simulink model "SingleStreamSSRwithPL"  (R2023a)
settings: Solver=VariableStepAuto  StartTime=0.0  StopTime=512  RelTol=1e-3
PreLoadFcn:
  | xmcCheckSlxPath(bdroot);
  | SSR4withPL_init;
InitFcn:
  | xmcCheckSlxPath(bdroot);
  | SSR4withPL_init;
undefined symbols (not defined in the file): c, FIR_MultiKernel_cin, FIR_MultiKernel_cincout, FIR_MultiKernel_cout, S, SHIFT_ACC, SingleStream, T, Taps, VectorSize, vsva2197, xcvc1902
libraries: hdlBasic x45, aieBasic x40, aieUtilities x32, hdlUtilities x24, dspsrcs4 x1, simulink x1, vmcUtilities x1
(part 3 of 3)

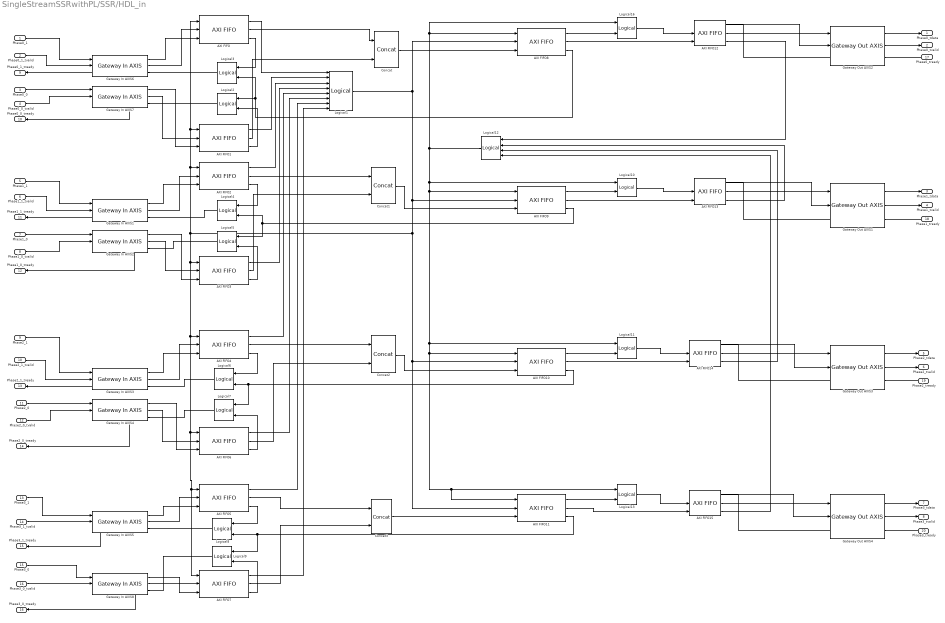
== system SingleStreamSSRwithPL/SSR/HDL_in ==
  Phase0_1 : Inport
  Phase0_1_tvalid : Inport  Port=2
  Phase0_0 : Inport  Port=3
  Phase0_0_tvalid : Inport  Port=4
  Phase1_1 : Inport  Port=5
  Phase1_1_tvalid : Inport  Port=6
  Phase1_0 : Inport  Port=7
  Phase1_0_tvalid : Inport  Port=8
  Phase2_1 : Inport  Port=9
  Phase2_1_tvalid : Inport  Port=10
  Phase2_0 : Inport  Port=11
  Phase2_0_tvalid : Inport  Port=12
  Phase3_1 : Inport  Port=13
  Phase3_1_tvalid : Inport  Port=14
  Phase3_0 : Inport  Port=15
  Phase3_0_tvalid : Inport  Port=16
  Phase0_tready : Inport  Port=17
  Phase1_tready : Inport  Port=18
  Phase2_tready : Inport  Port=19
  Phase3_tready : Inport  Port=20
  AXI FIFO{,1..15} (16 alike) : hdlBasic/AXI FIFO  input_depth_axis=1K  actual_fifo_depth_label=1026  enable_tdata=on  enable_tdest=off  enable_tstrb=off  enable_tready=on  enable_tid=off  enable_tuser=off  enable_tkeep=off  enable_tlast=off  has_aresetn=off  enable_data_counts_axis=off  fifo_implementation_type_axis=Common Clock Block RAM  trim_axipin_name=on  programmable_full_type_axis=Full  full_threshold_assert_value_axis=0  programmable_empty_type_axis=Empty  empty_threshold_assert_value_axis=1022  underflow_flag_axi=0  underflow_sense_axi=Active High  overflow_flag_axi=0  overflow_sense_axi=Active High  simulation_type=fast_sim  XmcBlockStatus=1  maskContainerNames=tabcontainer1  block_type=axi_fifo  block_config=sysgen:AXI_FIFO_config
  Concat{,1..3} (4 alike) : hdlBasic/Concat  num_inputs=2  XmcBlockStatus=1  maskContainerNames=group1  block_type=concat  block_config=sysgen:Concat_config
  Gateway In AXIS{1..8} (8 alike) : hdlUtilities/Gateway In AXIS  gui_display_data_type=Fixed-point  arith_type=Unsigned  n_bits=32  bin_pt=0  preci_type=Custom  exp_width=16  frac_width=24  quantization=Truncate  overflow=Flag as error  OutSampleTime=1  block_type=gatewayinaxi  XmcBlockStatus=1
  Gateway Out AXIS{1..4} (4 alike) : hdlUtilities/Gateway Out AXIS  mask_sample_period=1  block_type=gatewayoutaxi
  Logical1 : hdlBasic/Logical  logical_function=AND  inputs=8  en=off  latency=0  precision=Full  arith_type=Unsigned  n_bits=16  bin_pt=0  align_bp=on  overflow=[]  quantization=[]  XmcBlockStatus=1  maskContainerNames=tabcontainer1  block_type=logical  block_config=sysgen:Logical_config
  Logical{2..11,13,16} (12 alike) : hdlBasic/Logical  logical_function=AND  inputs=2  en=off  latency=0  precision=Full  arith_type=Unsigned  n_bits=16  bin_pt=0  align_bp=on  overflow=[]  quantization=[]  XmcBlockStatus=1  maskContainerNames=tabcontainer1  block_type=logical  block_config=sysgen:Logical_config
  Logical12 : hdlBasic/Logical  logical_function=AND  inputs=4  en=off  latency=0  precision=Full  arith_type=Unsigned  n_bits=16  bin_pt=0  align_bp=on  overflow=[]  quantization=[]  XmcBlockStatus=1  maskContainerNames=tabcontainer1  block_type=logical  block_config=sysgen:Logical_config
  Phase0_tdata : Outport
  Phase0_tvalid : Outport  Port=2
  Phase1_tdata : Outport  Port=3
  Phase1_tvalid : Outport  Port=4
  Phase2_tdata : Outport  Port=5
  Phase2_tvalid : Outport  Port=6
  Phase3_tdata : Outport  Port=7
  Phase3_tvalid : Outport  Port=8
  Phase0_1_tready : Outport  Port=9
  Phase0_0_tready : Outport  Port=10
  Phase1_1_tready : Outport  Port=11
  Phase1_0_tready : Outport  Port=12
  Phase2_1_tready : Outport  Port=13
  Phase2_0_tready : Outport  Port=14
  Phase3_1_tready : Outport  Port=15
  Phase3_0_tready : Outport  Port=16
  wires:
  Gateway Out AXIS2/1 -> Phase0_tdata/1
  Gateway Out AXIS2/2 -> Phase0_tvalid/1
  Gateway Out AXIS1/1 -> Phase1_tdata/1
  Gateway Out AXIS1/2 -> Phase1_tvalid/1
  Gateway Out AXIS3/2 -> Phase2_tvalid/1
  Gateway Out AXIS3/1 -> Phase2_tdata/1
  Gateway Out AXIS4/2 -> Phase3_tvalid/1
  Gateway Out AXIS4/1 -> Phase3_tdata/1
  Phase0_1/1 -> Gateway In AXIS6/1
  Gateway In AXIS6/3 -> Phase0_1_tready/1
  Phase0_0/1 -> Gateway In AXIS7/1
  Gateway In AXIS7/3 -> Phase0_0_tready/1
  Phase0_tready/1 -> Gateway Out AXIS2/3
  Gateway In AXIS6/1 -> AXI FIFO/3
  Gateway In AXIS7/1 -> AXI FIFO1/3
  Gateway In AXIS6/2 -> AXI FIFO/2
  Gateway In AXIS7/2 -> AXI FIFO1/2
  Concat/1 -> AXI FIFO8/3
  Phase1_1/1 -> Gateway In AXIS1/1
  Gateway In AXIS1/3 -> Phase1_1_tready/1
  Phase1_0/1 -> Gateway In AXIS2/1
  Gateway In AXIS2/3 -> Phase1_0_tready/1
  Phase1_tready/1 -> Gateway Out AXIS1/3
  Gateway In AXIS2/2 -> AXI FIFO3/2
  AXI FIFO3/2 -> Concat1/2
  Gateway In AXIS2/1 -> AXI FIFO3/3
  Gateway In AXIS1/2 -> AXI FIFO2/2
  AXI FIFO3/3 -> Logical5/2
  Gateway In AXIS1/1 -> AXI FIFO2/3
  AXI FIFO2/3 -> Logical4/1
  Phase2_1/1 -> Gateway In AXIS3/1
  Gateway In AXIS3/3 -> Phase2_1_tready/1
  Phase2_0/1 -> Gateway In AXIS4/1
  Gateway In AXIS4/3 -> Phase2_0_tready/1
  Phase2_tready/1 -> Gateway Out AXIS3/3
  Phase3_1/1 -> Gateway In AXIS5/1
  Gateway In AXIS5/3 -> Phase3_1_tready/1
  Phase3_0/1 -> Gateway In AXIS8/1
  Gateway In AXIS8/3 -> Phase3_0_tready/1
  Phase3_tready/1 -> Gateway Out AXIS4/3
  Gateway In AXIS3/1 -> AXI FIFO4/3
  Gateway In AXIS4/2 -> AXI FIFO6/2
  Gateway In AXIS3/2 -> AXI FIFO4/2
  Gateway In AXIS4/1 -> AXI FIFO6/3
  Gateway In AXIS8/1 -> AXI FIFO7/3
  Gateway In AXIS8/2 -> AXI FIFO7/2
  Gateway In AXIS5/2 -> AXI FIFO5/2
  Logical1/1 -> AXI FIFO/1, AXI FIFO1/1, AXI FIFO2/1, AXI FIFO3/1, AXI FIFO4/1, AXI FIFO6/1, AXI FIFO5/1, AXI FIFO7/1, AXI FIFO10/2, AXI FIFO11/2, AXI FIFO9/2, AXI FIFO8/2
  Gateway In AXIS5/1 -> AXI FIFO5/3
  AXI FIFO/1 -> Logical1/1
  AXI FIFO1/1 -> Logical1/2
  AXI FIFO2/1 -> Logical1/3
  AXI FIFO3/1 -> Logical1/4
  AXI FIFO4/1 -> Logical1/5
  AXI FIFO6/1 -> Logical1/6
  AXI FIFO5/1 -> Logical1/7
  AXI FIFO7/1 -> Logical1/8
  AXI FIFO2/2 -> Concat1/1
  AXI FIFO/2 -> Concat/1
  AXI FIFO1/2 -> Concat/2
  AXI FIFO4/2 -> Concat2/1
  AXI FIFO6/2 -> Concat2/2
  AXI FIFO5/2 -> Concat3/1
  AXI FIFO7/2 -> Concat3/2
  Phase0_1_tvalid/1 -> Gateway In AXIS6/2
  Phase0_0_tvalid/1 -> Gateway In AXIS7/2
  Phase1_1_tvalid/1 -> Gateway In AXIS1/2
  Phase1_0_tvalid/1 -> Gateway In AXIS2/2
  Phase2_1_tvalid/1 -> Gateway In AXIS3/2
  Phase2_0_tvalid/1 -> Gateway In AXIS4/2
  Phase3_1_tvalid/1 -> Gateway In AXIS5/2
  Phase3_0_tvalid/1 -> Gateway In AXIS8/2
  Logical3/1 -> Gateway In AXIS6/3
  AXI FIFO8/3 -> Logical3/2, Logical2/1
  AXI FIFO1/3 -> Logical2/2
  AXI FIFO/3 -> Logical3/1
  Logical2/1 -> Gateway In AXIS7/3
  Concat1/1 -> AXI FIFO9/3
  AXI FIFO9/3 -> Logical4/2, Logical5/1
  Logical4/1 -> Gateway In AXIS1/3
  Logical5/1 -> Gateway In AXIS2/3
  Concat2/1 -> AXI FIFO10/3
  AXI FIFO6/3 -> Logical7/2
  AXI FIFO4/3 -> Logical6/1
  AXI FIFO10/3 -> Logical7/1, Logical6/2
  Logical6/1 -> Gateway In AXIS3/3
  Logical7/1 -> Gateway In AXIS4/3
  AXI FIFO7/3 -> Logical9/2
  AXI FIFO5/3 -> Logical8/1
  AXI FIFO11/3 -> Logical9/1, Logical8/2
  Concat3/1 -> AXI FIFO11/3
  Logical8/1 -> Gateway In AXIS5/3
  Logical9/1 -> Gateway In AXIS8/3
  Logical10/1 -> AXI FIFO13/2
  AXI FIFO10/1 -> Logical11/2
  AXI FIFO11/1 -> Logical13/2
  Logical13/1 -> AXI FIFO15/2
  Logical16/1 -> AXI FIFO12/2
  Logical12/1 -> Logical16/1, AXI FIFO8/1, Logical10/1, Logical11/1, AXI FIFO10/1, Logical13/1, AXI FIFO11/1, AXI FIFO9/1
  AXI FIFO9/2 -> AXI FIFO13/3
  AXI FIFO10/2 -> AXI FIFO14/3
  AXI FIFO11/2 -> AXI FIFO15/3
  AXI FIFO12/3 -> Logical12/1
  AXI FIFO13/3 -> Logical12/2
  AXI FIFO14/3 -> Logical12/3
  AXI FIFO15/3 -> Logical12/4
  AXI FIFO8/2 -> AXI FIFO12/3
  AXI FIFO12/2 -> Gateway Out AXIS2/1
  AXI FIFO12/1 -> Gateway Out AXIS2/2
  Gateway Out AXIS2/3 -> AXI FIFO12/1
  Gateway Out AXIS1/3 -> AXI FIFO13/1
  AXI FIFO13/2 -> Gateway Out AXIS1/1
  AXI FIFO13/1 -> Gateway Out AXIS1/2
  Logical11/1 -> AXI FIFO14/2
  AXI FIFO14/1 -> Gateway Out AXIS3/2
  AXI FIFO14/2 -> Gateway Out AXIS3/1
  Gateway Out AXIS3/3 -> AXI FIFO14/1
  AXI FIFO15/2 -> Gateway Out AXIS4/1
  AXI FIFO15/1 -> Gateway Out AXIS4/2
  Gateway Out AXIS4/3 -> AXI FIFO15/1
  AXI FIFO9/1 -> Logical10/2
  AXI FIFO8/1 -> Logical16/2

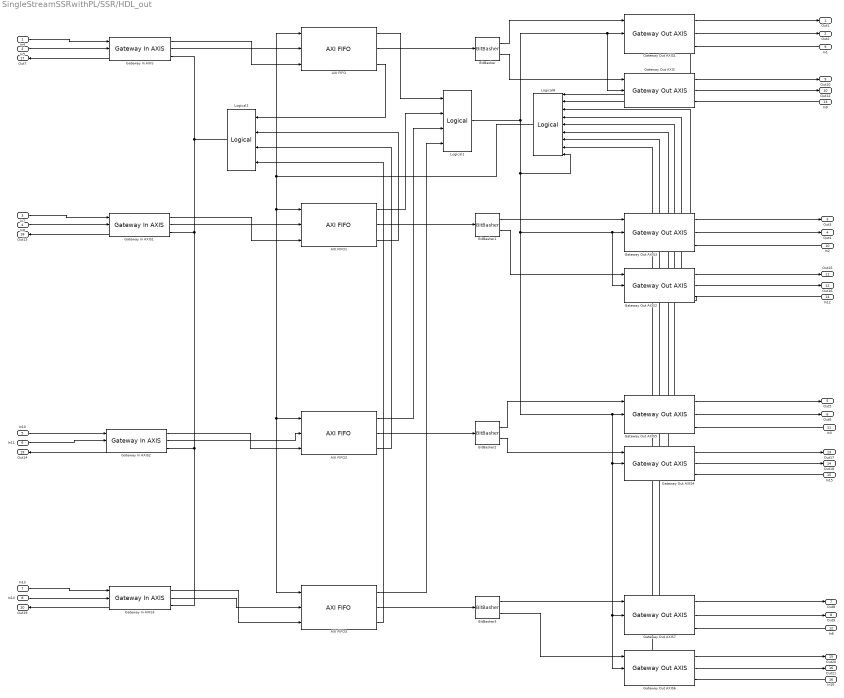
== system SingleStreamSSRwithPL/SSR/HDL_out ==
  In4 : Inport
  In5 : Inport  Port=2
  In7 : Inport  Port=3
  In8 : Inport  Port=4
  In10 : Inport  Port=5
  In11 : Inport  Port=6
  In13 : Inport  Port=7
  In14 : Inport  Port=8
  In1 : Inport  Port=9
  In2 : Inport  Port=10
  In3 : Inport  Port=11
  In6 : Inport  Port=12
  In9 : Inport  Port=13
  In12 : Inport  Port=14
  In15 : Inport  Port=15
  In16 : Inport  Port=16
  AXI FIFO{,1..3} (4 alike) : hdlBasic/AXI FIFO  input_depth_axis=32  actual_fifo_depth_label=34  enable_tdata=on  enable_tdest=off  enable_tstrb=off  enable_tready=on  enable_tid=off  enable_tuser=off  enable_tkeep=off  enable_tlast=off  has_aresetn=off  enable_data_counts_axis=off  fifo_implementation_type_axis=Common Clock Block RAM  trim_axipin_name=on  programmable_full_type_axis=Full  full_threshold_assert_value_axis=0  programmable_empty_type_axis=Empty  empty_threshold_assert_value_axis=1022  underflow_flag_axi=0  underflow_sense_axi=Active High  overflow_flag_axi=0  overflow_sense_axi=Active High  simulation_type=fast_sim  XmcBlockStatus=1  maskContainerNames=tabcontainer1  block_type=axi_fifo  block_config=sysgen:AXI_FIFO_config
  BitBasher : hdlBasic/BitBasher  bitexpr=|  display_expr=off  sr_1=lo  arith_type1=Unsigned  bin_pt1=0  sr_2=hi  arith_type2=Unsigned  bin_pt2=0  sr_3=3  arith_type3=Unsigned  bin_pt3=0  sr_4=4  arith_type4=Unsigned  bin_pt4=0  XmcBlockStatus=1  maskContainerNames=group1  block_type=bitbasher  block_config=sysgen:BitBasher_config
      | lo={in[31:0]}
      | hi={in[63:32]}
  BitBasher1 : hdlBasic/BitBasher  bitexpr=|  display_expr=off  sr_1=lo  arith_type1=Unsigned  bin_pt1=0  sr_2=hi  arith_type2=Unsigned  bin_pt2=0  sr_3=3  arith_type3=Unsigned  bin_pt3=0  sr_4=4  arith_type4=Unsigned  bin_pt4=0  XmcBlockStatus=1  maskContainerNames=group1  block_type=bitbasher  block_config=sysgen:BitBasher_config
      | lo={in[31:0]}
      | hi={in[63:32]}
  BitBasher2 : hdlBasic/BitBasher  bitexpr=|  display_expr=off  sr_1=lo  arith_type1=Unsigned  bin_pt1=0  sr_2=hi  arith_type2=Unsigned  bin_pt2=0  sr_3=3  arith_type3=Unsigned  bin_pt3=0  sr_4=4  arith_type4=Unsigned  bin_pt4=0  XmcBlockStatus=1  maskContainerNames=group1  block_type=bitbasher  block_config=sysgen:BitBasher_config
      | lo={in[31:0]}
      | hi={in[63:32]}
  BitBasher3 : hdlBasic/BitBasher  bitexpr=|  display_expr=off  sr_1=lo  arith_type1=Unsigned  bin_pt1=0  sr_2=hi  arith_type2=Unsigned  bin_pt2=0  sr_3=3  arith_type3=Unsigned  bin_pt3=0  sr_4=4  arith_type4=Unsigned  bin_pt4=0  XmcBlockStatus=1  maskContainerNames=group1  block_type=bitbasher  block_config=sysgen:BitBasher_config
      | lo={in[31:0]}
      | hi={in[63:32]}
  Gateway In AXIS{,1..3} (4 alike) : hdlUtilities/Gateway In AXIS  gui_display_data_type=Fixed-point  arith_type=Unsigned  n_bits=64  bin_pt=0  preci_type=Custom  exp_width=16  frac_width=24  quantization=Truncate  overflow=Flag as error  OutSampleTime=1  block_type=gatewayinaxi  XmcBlockStatus=1
  Gateway Out AXIS{,1..7} (8 alike) : hdlUtilities/Gateway Out AXIS  mask_sample_period=1  block_type=gatewayoutaxi
  Logical1 : hdlBasic/Logical  logical_function=AND  inputs=4  en=off  latency=0  precision=Full  arith_type=Unsigned  n_bits=16  bin_pt=0  align_bp=on  overflow=[]  quantization=[]  XmcBlockStatus=1  maskContainerNames=tabcontainer1  block_type=logical  block_config=sysgen:Logical_config
  Logical2 : hdlBasic/Logical  logical_function=AND  inputs=4  en=off  latency=0  precision=Full  arith_type=Unsigned  n_bits=16  bin_pt=0  align_bp=on  overflow=[]  quantization=[]  XmcBlockStatus=1  maskContainerNames=tabcontainer1  block_type=logical  block_config=sysgen:Logical_config
  Logical8 : hdlBasic/Logical  logical_function=AND  inputs=9  en=off  latency=0  precision=Full  arith_type=Unsigned  n_bits=16  bin_pt=0  align_bp=on  overflow=[]  quantization=[]  XmcBlockStatus=1  maskContainerNames=tabcontainer1  block_type=logical  block_config=sysgen:Logical_config
  Out1 : Outport
  Out2 : Outport  Port=2
  Out3 : Outport  Port=3
  Out4 : Outport  Port=4
  Out5 : Outport  Port=5
  Out6 : Outport  Port=6
  Out8 : Outport  Port=7
  Out9 : Outport  Port=8
  Out10 : Outport  Port=9
  Out12 : Outport  Port=10
  Out15 : Outport  Port=11
  Out16 : Outport  Port=12
  Out17 : Outport  Port=13
  Out18 : Outport  Port=14
  Out20 : Outport  Port=15
  Out21 : Outport  Port=16
  Out7 : Outport  Port=17
  Out13 : Outport  Port=18
  Out14 : Outport  Port=19
  Out19 : Outport  Port=20
  wires:
  Gateway Out AXIS5/2 -> Out6/1
  Gateway Out AXIS7/1 -> Out8/1
  Gateway Out AXIS7/2 -> Out9/1
  AXI FIFO/3 -> Logical2/1
  BitBasher1/1 -> Gateway Out AXIS3/1
  In16/1 -> Gateway Out AXIS6/3
  BitBasher2/1 -> Gateway Out AXIS5/1
  Gateway In AXIS/3 -> Out7/1
  In10/1 -> Gateway In AXIS2/1
  In11/1 -> Gateway In AXIS2/2
  In3/1 -> Gateway Out AXIS5/3
  Gateway Out AXIS2/1 -> Out15/1
  Gateway In AXIS1/1 -> AXI FIFO1/3
  Gateway In AXIS2/2 -> AXI FIFO2/2
  Gateway In AXIS3/2 -> AXI FIFO3/2
  BitBasher3/1 -> Gateway Out AXIS7/1
  BitBasher2/2 -> Gateway Out AXIS4/1
  In1/1 -> Gateway Out AXIS1/3
  Gateway In AXIS2/3 -> Out14/1
  Gateway In AXIS/2 -> AXI FIFO/2
  AXI FIFO1/1 -> Logical1/2
  Gateway In AXIS2/1 -> AXI FIFO2/3
  AXI FIFO/2 -> BitBasher/1
  In8/1 -> Gateway In AXIS1/2
  Gateway In AXIS/1 -> AXI FIFO/3
  In5/1 -> Gateway In AXIS/2
  Gateway Out AXIS5/3 -> Logical8/5
  In7/1 -> Gateway In AXIS1/1
  In9/1 -> Gateway Out AXIS/3
  In14/1 -> Gateway In AXIS3/2
  AXI FIFO2/1 -> Logical1/3
  Gateway Out AXIS1/1 -> Out1/1
  Gateway Out AXIS4/2 -> Out18/1
  AXI FIFO2/3 -> Logical2/3
  Gateway Out AXIS/1 -> Out10/1
  Gateway Out AXIS6/2 -> Out21/1
  In12/1 -> Gateway Out AXIS2/3
  Gateway Out AXIS/2 -> Out12/1
  AXI FIFO1/2 -> BitBasher1/1
  Gateway Out AXIS3/1 -> Out3/1
  Gateway Out AXIS5/1 -> Out5/1
  Gateway In AXIS3/1 -> AXI FIFO3/3
  BitBasher1/2 -> Gateway Out AXIS2/1
  Gateway Out AXIS/3 -> Logical8/2
  BitBasher/2 -> Gateway Out AXIS/1
  In15/1 -> Gateway Out AXIS4/3
  AXI FIFO3/1 -> Logical1/4
  Gateway Out AXIS3/2 -> Out4/1
  Gateway Out AXIS6/1 -> Out20/1
  In4/1 -> Gateway In AXIS/1
  Gateway In AXIS3/3 -> Out19/1
  Gateway Out AXIS2/2 -> Out16/1
  AXI FIFO3/2 -> BitBasher3/1
  Gateway In AXIS1/3 -> Out13/1
  Gateway Out AXIS6/3 -> Logical8/8
  Gateway Out AXIS4/1 -> Out17/1
  Logical2/1 -> Gateway In AXIS2/3, Gateway In AXIS3/3, Gateway In AXIS1/3, Gateway In AXIS/3
  Logical8/1 -> AXI FIFO1/1, AXI FIFO2/1, AXI FIFO3/1, AXI FIFO/1
  In2/1 -> Gateway Out AXIS3/3
  Gateway Out AXIS2/3 -> Logical8/4
  AXI FIFO/1 -> Logical1/1
  Gateway In AXIS1/2 -> AXI FIFO1/2
  Gateway Out AXIS3/3 -> Logical8/3
  In13/1 -> Gateway In AXIS3/1
  Logical1/1 -> Gateway Out AXIS/2, Gateway Out AXIS1/2, Gateway Out AXIS7/2, Gateway Out AXIS6/2, Gateway Out AXIS4/2, Gateway Out AXIS5/2, Gateway Out AXIS2/2, Gateway Out AXIS3/2, Logical8/9
  Gateway Out AXIS4/3 -> Logical8/6
  Gateway Out AXIS1/2 -> Out2/1
  Gateway Out AXIS7/3 -> Logical8/7
  AXI FIFO3/3 -> Logical2/4
  Gateway Out AXIS1/3 -> Logical8/1
  BitBasher3/2 -> Gateway Out AXIS6/1
  In6/1 -> Gateway Out AXIS7/3
  AXI FIFO1/3 -> Logical2/2
  BitBasher/1 -> Gateway Out AXIS1/1
  AXI FIFO2/2 -> BitBasher2/1

== matlab function SingleStreamSSRwithPL/ComplexSource/MATLAB Function ==
  data: u input; y1 output; y2 output; y3 output; y4 output; y5 output; y6 output; y7 output; y8 output
function [y1,y2,y3,y4,y5,y6,y7,y8] = fcn(u)


y1 = u(1:8:end);
y2 = u(2:8:end);
y3 = u(3:8:end);
y4 = u(4:8:end);
y5 = u(5:8:end);
y6 = u(6:8:end);
y7 = u(7:8:end);
y8 = u(8:8:end);
